simulink model "Genset"  (R2022a)
settings: Solver=VariableStepAuto  StartTime=0.0  StopTime=10  RelTol=1e-3
undefined symbols (not defined in the file): p
libraries: simulink x2
settings Model: Creator=a.dehghan  LastModifiedBy=a.dehghan

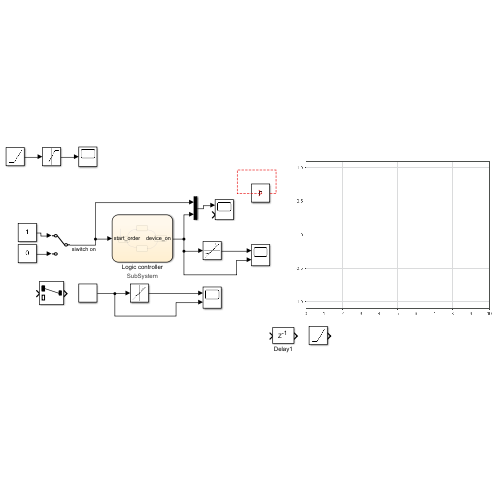
[thumbnail: Simulink's stored preview of the top-level diagram]
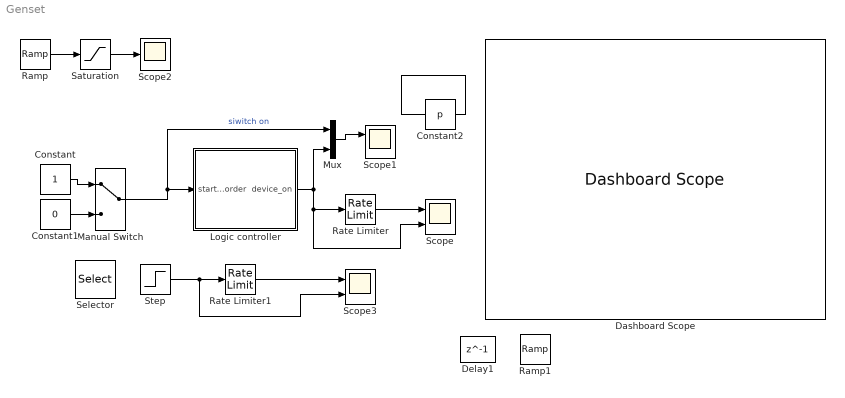
== system Genset ==
  Constant : Constant
  Constant1 : Constant  Value=0
  Constant2 : Constant  Value=p
  Dashboard Scope : DashboardScope
  Delay1 : Delay  DelayLength=1  InitialCondition=0  UseCircularBuffer=on
  Logic controller : Stateflow chart  Description=vhk,ncg,vbh,v  TreatAsAtomicUnit=on
      settings: AttributesFormatString=%<BlockType>
  Manual Switch : ManualSwitch
  Mux : Mux  Inputs=2
  Ramp : simulink/Sources/Ramp  slope=1  start=600  InitialOutput=0
  Ramp1 : simulink/Sources/Ramp  slope=0.05  start=600  InitialOutput=0
  Rate Limiter : RateLimiter  RisingSlewLimit=2  FallingSlewLimit=-10  SampleTimeMode=inherited
  Rate Limiter1 : RateLimiter  RisingSlewLimit=0.5  FallingSlewLimit=-10  SampleTimeMode=inherited
  Saturation : Saturate  UpperLimit=200  LowerLimit=0
  Scope : Scope  NumInputPorts=2
  Scope1 : Scope  NumInputPorts=2
  Scope2 : Scope
  Scope3 : Scope  NumInputPorts=2
  Selector : Selector  InputPortWidth=2  IndexOptions=Index vector (dialog)  Indices=[1]  OutputSizes=1
  Step : Step  SampleTime=0
  wires:
  Ramp/1 -> Saturation/1
  Constant/1 -> Manual Switch/1
  Constant1/1 -> Manual Switch/2
  Manual Switch/1 -> Mux/1, Logic controller/1(start_order)  "siwitch on"
  Mux/1 -> Scope1/1
  Logic controller/1(device_on) -> Rate Limiter/1, Scope/2, Mux/2
  Rate Limiter/1 -> Scope/1
  Constant2/1 -> ?
  Saturation/1 -> Scope2/1
  Step/1 -> Scope3/2, Rate Limiter1/1
  Rate Limiter1/1 -> Scope3/1

== stateflow chart Genset/Logic controller ==
  state start_transition
    entry :
  state on
    entry : device_on = 1;
  state off
    entry : device_on = 0;
  state stop_transition
  (default) -> off
  off -> start_transition : [start_order == 1]
  start_transition -> on : after(600,sec)
  on -> stop_transition : [start_order == 0]
  stop_transition -> off : after(1800,sec)
  data: device_on output; start_order input
